simulink model "Rus_ver_model"  (R2021b)
settings: Solver=ode15s  StartTime=0.0  StopTime=10  FixedStep=1e-2  MaxStep=tsTraj  RelTol=1e-3  EnableMultiTasking=on
values from neighbouring files (symbols this model uses):
  bd_spine_damping = 0    [CostFcnPDcontroll.m]    (also in CostFuncOptimizeSpine.m = spine_param(3); last_scores.mat = 10)
  bd_spine_eq_pos = 0    [CostFcnPDcontroll.m]    (also in CostFuncOptimizeSpine.m = deg2rad(spine_param(1)); last_scores.mat)
  bd_spine_stiffness = 0    [CostFcnPDcontroll.m]    (also in CostFuncOptimizeSpine.m = spine_param(2); last_scores.mat = 300)
  body_dim = [0.267 0.194 0.114]    [last_scores.mat]    (also in robotParameters.m)
  body_mass = 6.0    (= 6)    [CostOfTransport.m]    (also in last_scores.mat; robotParameters.m)
  delta_gait_front = delays(1)    [CostFuncOptimizeSpine.m]    (also in PD_optimizedData_16Mar22_1632.mat = 48; PD_optimizedData_16Mar22_2228_good.mat = 58; PD_optimizedData_17Mar22_1432_vel_walk_03735.mat = 56; PD_optimizedData_18Mar22_1518_right_direction.mat = 46)
  delta_gait_rear = delays(2)    [CostFuncOptimizeSpine.m]    (also in PD_optimizedData_16Mar22_1632.mat = 56; PD_optimizedData_16Mar22_2228_good.mat = 40; PD_optimizedData_17Mar22_1432_vel_walk_03735.mat = 6; PD_optimizedData_18Mar22_1518_right_direction.mat = 76)
  fem_der_front = [0 1.0471975512 -3.66519142919 -6.45771823238 -0.523598775598 5.41052068118 0]    [last_scores.mat]
  fem_der_rear = [0 -2.61799387799 -0.872664625997 1.2217304764 4.88692190558 1.3962634016 0]    [last_scores.mat]
  fem_motionFront = femur_motionFront    [CostFcnPDcontroll.m]    (also in CostFuncOptimizeSpine.m = deg2rad([params(1:N), params(1)]); getFiguresAngOmTau.m; last_scores.mat = [-2.12930168743 -2.33874119767 -2.26892802759 -2.12930168743; nonlinearContraints.m = deg2rad([x(1:N), x(1)]))
  fem_motionRear = femur_motionRear    [CostFcnPDcontroll.m]    (also in CostFuncOptimizeSpine.m = deg2rad([params(2*N+1:3*N), params(2*N+1)]); getFiguresAngOmTau.m; last_scores.mat = [-2.09439510239 -2.12930168743 -2.16420827247 -2.19911485751; nonlinearContraints.m = deg2rad([x(2*N+1:3*N), x(2*N+1)]))
  gait_period = 1.2    [PD_optimizedData_16Mar22_1632.mat]    (also in PD_optimizedData_16Mar22_2228_good.mat; PD_optimizedData_17Mar22_1432_vel_walk_03735.mat; PD_optimizedData_18Mar22_1518_right_direction.mat; PD_optimizedData_18Mar22_1539.mat)
  ground = [20 2 0.1]    [last_scores.mat]    (also in robotParameters.m = [20 1.5 0.05])
  hip_mass = 0.595    [CostOfTransport.m]    (also in last_scores.mat; robotParameters.m)
  hip_radius = 0.046    [last_scores.mat]    (also in robotParameters.m)
  max_torque = 33.5    [last_scores.mat]    (also in robotParameters.m)
  N = (numel(params)-5)/4    [CostFuncOptimizeSpine.m]    (also in nonlinearContraints.m = (numel(x)-2)/4; nonlinearContraintsSpine.m = (numel(x)-5)/4; pampam.m = numel(params)/2)
  tib_der_front = [0 -1.74532925199 0.349065850399 0 1.57079632679 1.74532925199 0]    [last_scores.mat]
  tib_der_rear = [0 0.698131700798 -1.3962634016 3.31612557879 2.44346095279 -4.01425727959 0]    [last_scores.mat]
  tib_motionFront = tibia_motionFront    [CostFcnPDcontroll.m]    (also in CostFuncOptimizeSpine.m = deg2rad([params(N+1:2*N), params(N+1)]); getFiguresAngOmTau.m; last_scores.mat = [1.0471975512 0.977384381117 0.872664625997 0.977384381117 1; nonlinearContraints.m = deg2rad([x(N+1:2*N), x(N+1)]))
  tib_motionRear = tibia_motionRear    [CostFcnPDcontroll.m]    (also in CostFuncOptimizeSpine.m = deg2rad([params(3*N+1:4*N), params(3*N+1)]); getFiguresAngOmTau.m; last_scores.mat = [0.942477796077 1.08210413624 0.733038285838 1.18682389136 1; nonlinearContraints.m = deg2rad([x(3*N+1:4*N), x(3*N+1)]))
  traj_times = linspace(0,gait_period,N+1)    [CostFuncOptimizeSpine.m]    (also in PD_optimizedData_16Mar22_1632.mat = [0 0.2 0.4 0.6 0.8 1 1.2]; PD_optimizedData_16Mar22_2228_good.mat = [0 0.2 0.4 0.6 0.8 1 1.2]; PD_optimizedData_17Mar22_1432_vel_walk_03735.mat = [0 0.2 0.4 0.6 0.8 1 1.2]; PD_optimizedData_18Mar22_1518_right_direction.mat = [0 0.2 0.4 0.6 0.8 1 1.2])
  tsTraj = 0.01    [last_scores.mat]    (also in pampam.m; robotParameters.m)
undefined symbols (not defined in the file or in its folder): X, Y, Z
libraries: sm_lib x72, simulink x12, nesl_utility x10, robotcorelib x4, QR_leg_rus_ver x4
(part 1 of 3)
settings Model: SimulationMode=accelerator  Creator=boris_1863  LastModifiedBy=YEfim
settings SolverCC: AlgebraicLoopSolver=TrustRegion  SolverResetMethod=Robust
settings DataIOCC: LimitDataPoints=on  MaxDataPoints=10000
settings OptimizationCC: LifeSpan=inf
settings DebuggingCC: IgnoredZcDiagnostic=none  AllowSymbolicDim=off  SFUnexpectedBacktrackingDiag=warning  SFNoUnconditionalDefaultTransitionDiag=warning  SFExecutionAtInitializationDiag=none  SFMachineParentedDataDiag=warning  ArithmeticOperatorsInVariantConditions=warning
settings HardwareCC: ProdBitPerLong=64  ProdHWDeviceType=Intel->x86-64 (Linux 64)
settings SFSimCC: SimUseLocalCustomCode=off  CustomCodeUndefinedFunction=UseInterfaceOnly
settings RTWCC: RTWUseLocalCustomCode=off
settings CodeAppCC: StateflowObjectComments=on
settings GRTTargetCC: TargetLangStandard=C89/C90 (ANSI)
settings ConfigComp: CovMetricSettings=dw  CovSaveCumulativeToWorkspaceVar=on  CovSaveSingleToWorkspaceVar=on  CovExternalEMLEnable=off  CovSFcnEnable=off
settings SimscapeCC: SimscapeNormalizeSystem=off  SimscapeLogDataHistory=10000
settings DiagnosticsConfigSet: SimMechanicsInvalidVisualProperty=none  SimMechanicsCrossSectionNullEdge=none  SimMechanicsUnconnectedFramePorts=none  SimMechanicsUnconnectedGeometryPorts=none  SimMechanicsRedundantBlock=none  SimMechanicsConflictingReferenceFrames=none  SimMechanicsRigidlyBoundBlock=none  SimMechanicsUnsatisfiedHighPriorityTargets=none  SimMechanicsJointTargetOverSpecification=none
settings ExplorerConfigSet: InternalSimMechanicsExplorerSettings="<ExplorerConfiguration><canonicalview>default</canonicalview><AnimationSetting><BasePlaybackSpeed>1.0</BasePlaybackSpeed><PlaybackSpeedFactor>0.5</PlaybackSpeedFactor></AnimationSetting><TilePanel><TileInfo><Tiles Columns=\"1\" Count=\"1\" Rows=\"1\"><Column Weight=\"1\"/><Row Weight=\"1\"/><Tile Height=\"1\" Width=\"1\" X=\"0\" Y=\"0\"/></Tiles></TileInfo><SceneInfo><SceneViewer><BGColor><R>1</R><G>1</G><B>1</B></BGColor><Camera><DoPerspective>off</DoPerspective><Position><X>2.30591075274786395</X><Y>-10.1183993179019129</Y><Z>0.217589827418119802</Z></Position><Center><X>2.30591075274786395</X><Y>3.02154239351093423e-07</Y><Z>0.217589827418119802</Z></Center><Up><X>0</X><Y>-0</Y><Z>1</Z></Up><ViewLimDist>1</ViewLimDist><YLim>0.757338786635555206</YLim><XLim>2.71140067704754673</XLim></Camera></SceneViewer></SceneInfo></TilePanel><MechEditorPanel><Cameras/><GfxPanelCameraMap/><VideoCreator><PlaybackSpeedRatio>1.0</PlaybackSpeedRatio><FrameRate>60</FrameRate><VideoFormat>Motion JPEG AVI</VideoFormat><FrameSize>auto</FrameSize></VideoCreator></MechEditorPanel></ExplorerConfiguration>"

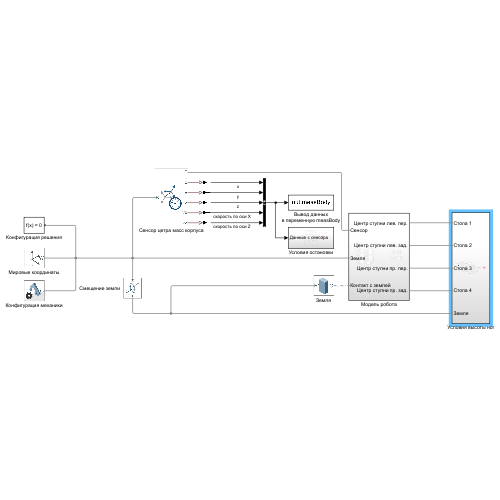
[thumbnail: Simulink's stored preview of the top-level diagram]
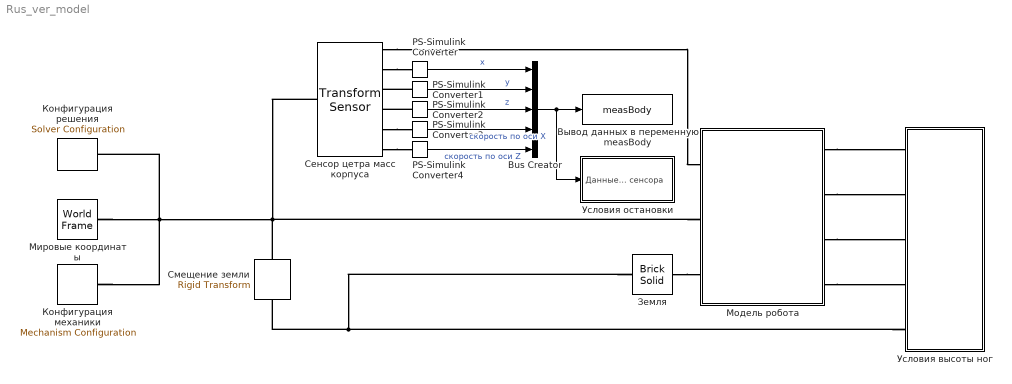
== system Rus_ver_model ==
  Bus Creator : BusCreator  Inputs=5
  PS-Simulink Converter : nesl_utility/PS-Simulink Converter  PhysicalDomain=network_engine_domain  SubClassName=ps_output  LeftPortType=input  RightPortType=output  PseudoPeriodic=off  Frequencies=[]  Unit=m  AffineConversion=off
      settings: SourceProductBaseCode=PW,SS
  PS-Simulink Converter1 : nesl_utility/PS-Simulink Converter  PhysicalDomain=network_engine_domain  SubClassName=ps_output  LeftPortType=input  RightPortType=output  PseudoPeriodic=off  Frequencies=[]  Unit=m  AffineConversion=off
      settings: SourceProductBaseCode=PW,SS
  PS-Simulink Converter2 : nesl_utility/PS-Simulink Converter  PhysicalDomain=network_engine_domain  SubClassName=ps_output  LeftPortType=input  RightPortType=output  PseudoPeriodic=off  Frequencies=[]  Unit=m  AffineConversion=off
      settings: SourceProductBaseCode=PW,SS
  PS-Simulink Converter3 : nesl_utility/PS-Simulink Converter  PhysicalDomain=network_engine_domain  SubClassName=ps_output  LeftPortType=input  RightPortType=output  PseudoPeriodic=off  Frequencies=[]  Unit=m/s  AffineConversion=off
      settings: SourceProductBaseCode=PW,SS
  PS-Simulink Converter4 : nesl_utility/PS-Simulink Converter  PhysicalDomain=network_engine_domain  SubClassName=ps_output  LeftPortType=input  RightPortType=output  PseudoPeriodic=off  Frequencies=[]  Unit=m/s  AffineConversion=off
      settings: SourceProductBaseCode=PW,SS
  Вывод данных в переменную measBody : ToWorkspace  VariableName=measBody  SaveFormat=Timeseries  SampleTime=-1
  Земля : sm_lib/Body Elements/Brick Solid  GraphicAmbientColor=[0.15 0.15 0.15 1.0]  BasedOnType=Density  BrickDimensions=ground  BrickDimensionUnits=m  CenterOfMass=[0 0 0]  CenterOfMassUnits=m  GraphicDiffuseColor=[0.5 0.5 0.5]  Density=1000  DensityUnits=kg/m^3  DoExposeReferenceFrame=off  GraphicEmissiveColor=[0.0 0.0 0.0 1.0]  ExportEntireGeometry=on  SerializedFrames=<Frames><Frame><Id>Frame1</Id><Value><Name>F1</Name><Origin><Source>GeometricFeature</Source><FeatureName>+z surface</FeatureName></Origin><PrimaryAxis><DefinedDirection>+Z</DefinedDirection><Source>ReferenceFrame</Source><SourceDirection>+Z</SourceDirection><FeatureName></FeatureName></PrimaryAxis><SecondaryAxis><DefinedDirection>+X</DefinedDirection><Source>ReferenceFrame</Source><SourceDirection>+X</SourceDirection><FeatureName></FeatureName></SecondaryAxis></Value></Frame></Frames>  MarkerShape=Sphere  MarkerSize=10  GraphicType=FromGeometry  InertiaType=CalculateFromGeometry  Mass=1  MassUnits=kg  MomentsOfInertia=[1 1 1]  MomentsOfInertiaUnits=kg*m^2  GraphicOpacity=1.0  ProductsOfInertia=[0 0 0]  ProductsOfInertiaUnits=kg*m^2  GraphicShininess=75  GraphicSpecularColor=[0.5 0.5 0.5 1.0]  GraphicVisPropType=SimpleVisualProperties
  Конфигурация механики : sm_lib/Utilities/Mechanism Configuration  UniformGravity=Constant  GravityVector=[0 0 -9.80665]  GravityUnits=m/s^2  LinearizationDelta=0.001  JointModeTransitionNonlinearIterations=2
  Конфигурация решения : nesl_utility/Solver Configuration  PhysicalDomain=network_engine_domain  SubClassName=solver  LeftPortType=input  RightPortType=generic  Tones=[]  Harmonics=[]  SimulateNoise=off  Profile=off  UseLocalSampling=off  EnableSwitchedLinearOptims=on  FrequencyDomain=off  UseCCode=off  RelTol=0.001  AbsTol=1e-06  MinStep=1e-09  ToWorkspace=off  RevertToSquareIcSolve=off  NumHomotopyIterations=100  PhasorMode=off  PhasorModeNumHarmonics=1  DoDC=off  ResidualTolerance=1e-09  UseLocalSolver=off  LocalSolverChoice=NE_BACKWARD_EULER_ADVANCER  LocalSolverSampleTime=0.001  DoFixedCost=off  MaxNonlinIter=3  MaxModeIter=2  ComputeImpulses=off  ImpulseIterations=2  LinearAlgebra=Sparse  EquationFormulation=NE_TIME_EF  DelaysMemoryBudget=1024  AutomaticFiltering=on  FilteringTimeConstant=0.001  PartitionStorageMethod=AS_NEEDED  PartitionMemoryBudget=1024  PartitionMethod=FAST
      settings: SourceProductBaseCode=PW,SS
  Мировые координаты : sm_lib/Frames and Transforms/World Frame
  Модель робота : Subsystem
  Сенсор цетра масс корпуса : sm_lib/Frames and Transforms/Transform Sensor  MeasurementFrame=World  SenseAngle=off  SenseAxis=off  SenseAngle1=off  SenseAngle2=off  SenseAngle3=off  SenseQ=off  SenseR=off  SenseOmegaX=off  SenseOmegaY=off  SenseOmegaZ=off  SenseOmega1=off  SenseOmega2=off  SenseOmega3=off  SenseQDot=off  SenseRDot=off  SenseAlphaX=off  SenseAlphaY=off  SenseAlphaZ=off  SenseAlpha1=off  SenseAlpha2=off  SenseAlpha3=off  SenseQDDot=off  SenseRDDot=off  SenseX=on  SenseY=on  SenseZ=on  SenseRad=off  SenseAzim=off  SenseDist=off  SenseInc=off  SenseXDot=on  SenseYDot=off  SenseZDot=on  SenseRadDot=off  SenseAzimDot=off  SenseDistDot=off  SenseIncDot=off  SenseXDDot=off  SenseYDDot=off  SenseZDDot=off  SenseRadDDot=off  SenseAzimDDot=off  SenseDistDDot=off  SenseIncDDot=off
  Смещение земли : sm_lib/Frames and Transforms/Rigid Transform  TranslationMethod=StandardAxis  TranslationStandardOffset=ground(1)/2-2  TranslationLengthUnit=m  TranslationStandardAxis=+X  TranslationCartesianOffset=[0 0 0]  TranslationROffset=0  TranslationROffsetUnits=m  TranslationZOffset=0  TranslationZOffsetUnits=m  TranslationThetaOffset=0  TranslationThetaOffsetUnits=deg  RotationMethod=None  RotationAngleUnits=deg  RotationStandardAxis=+Z  RotationAngle=0.0  RotationArbitraryAxis=[0 0 1]  FollAlignAxisA=+X  BaseAlignAxisA=+Y  FollAlignAxisB=+Y  BaseAlignAxisB=+Z  RotationSequenceAxes=FollowerAxes  RotationSequence=XYX  RotationSequenceAngles=[0 0 0]  RotationSequenceAnglesUnits=deg  RotationMatrix=[1 0 0; 0 1 0; 0 0 1]
  Условия высоты ног : Subsystem
  Условия остановки : Subsystem
  wires:
  PS-Simulink Converter/1 -> Bus Creator/1  "x"
  PS-Simulink Converter1/1 -> Bus Creator/2  "y"
  PS-Simulink Converter2/1 -> Bus Creator/3  "z"
  Bus Creator/1 -> Вывод данных в переменную measBody/1, Условия остановки/1(Данные с сенсора)
  PS-Simulink Converter3/1 -> Bus Creator/4  "скорость по оси X"
  PS-Simulink Converter4/1 -> Bus Creator/5  "скорость по оси Z"
  connections:
  Мировые координаты/RConn1 -- Конфигурация решения/RConn1 -- Сенсор цетра масс корпуса/LConn1 -- Смещение земли/LConn1 -- Модель робота/LConn2 -- Конфигурация механики/RConn1
  Земля/LConn1 -- Условия высоты ног/RConn5 -- Смещение земли/RConn1
  Сенсор цетра масс корпуса/RConn1 -- Модель робота/LConn1
  Земля/RConn1 -- Модель робота/LConn3
  Модель робота/RConn1 -- Условия высоты ног/RConn1
  Модель робота/RConn2 -- Условия высоты ног/RConn2
  Модель робота/RConn3 -- Условия высоты ног/RConn3
  Модель робота/RConn4 -- Условия высоты ног/RConn4
  Сенсор цетра масс корпуса/RConn2 -- PS-Simulink Converter/LConn1
  PS-Simulink Converter1/LConn1 -- Сенсор цетра масс корпуса/RConn3
  PS-Simulink Converter2/LConn1 -- Сенсор цетра масс корпуса/RConn4
  Сенсор цетра масс корпуса/RConn5 -- PS-Simulink Converter3/LConn1
  Сенсор цетра масс корпуса/RConn6 -- PS-Simulink Converter4/LConn1

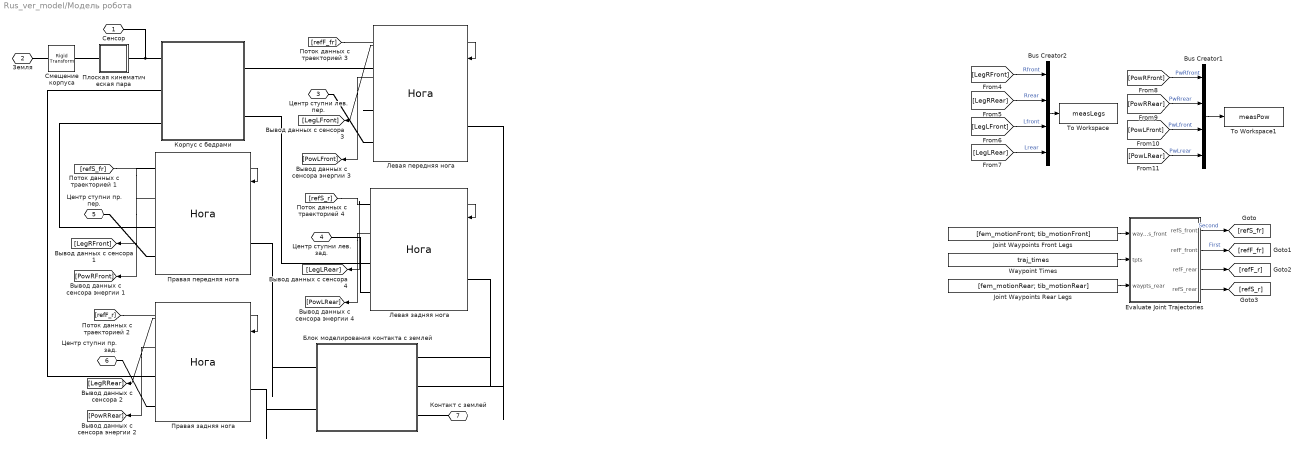
== system Rus_ver_model/Модель робота ==
  Bus Creator1 : BusCreator  Inputs=4
  Bus Creator2 : BusCreator  Inputs=4
  Evaluate Joint Trajectories : Subsystem
  Joint Waypoints Front Legs : Constant  Value=[fem_motionFront; tib_motionFront]
  Joint Waypoints Rear Legs : Constant  Value=[fem_motionRear; tib_motionRear]
  To Workspace : ToWorkspace  VariableName=measLegs  SaveFormat=Timeseries  SampleTime=-1
  To Workspace1 : ToWorkspace  VariableName=measPow  SaveFormat=Timeseries  SampleTime=-1
  Waypoint Times : Constant  Value=traj_times
  Блок моделирования контакта с землей : Subsystem
      settings: PortSchema="{\"entries\":[{\"content\":{\"sides\":[{\"content\":{\"connectorIds\":[]},\"type\":\"ConnectorPlacement.EquallySpacedRectSide\",\"uuid\":\"69850bd1-3a1b-4e19-820a-6c4fb91f3aa2\"},{\"content\":{\"connectorIds\":[],\"side\":\"RIGHT\"},\"type\":\"ConnectorPlacement.EquallySpacedRectSide\",\"uuid\":\"42ed8d47-3271-4e69-91e2-9f0454d59b48\"},{\"content\":{\"connectorIds\":[\"LConn1\",\"LConn2\"],\"side\":\"TOP\"},\"type\":\"ConnectorPlacement.EquallySpacedRectSide\",\"uuid\":\"114d7e17-c6c5-438c-9cb4-0dcf13920f6f\"},{\"content\":{\"connectorIds\":[\"RConn1\",\"RConn2\",\"RConn3\"],\"side\":\"BOTTOM\"},\"type\":\"ConnectorPlacement.EquallySpacedRectSide\",\"uuid\":\"caba5647-a516-4a04-8cbe-0248367597c4\"}]},\"type\":\"ConnectorPlacement.EquallySpacedConnector\",\"uuid\":\"24d64392-cc0c-4894-a6df-54d1d4435d86\"}],\"packageUris\":[\"http://schema.mathworks.com/mf0/Connector/R2020b\"],\"version\":\"1.0\"}"
  Корпус с бедрами : Subsystem  Variant=on  VariantControl=Choice  mask{spine_eq_pos=bd_spine_eq_pos, spine_stiffness=bd_spine_stiffness, spine_damping=bd_spine_damping}
      mask prompts: spine_eq_pos "Equilibrium Position"; spine_stiffness "Spring Stifness"; spine_damping "Damping Coefficient"
      mask DialogControl ParameterGroupVar Prompt: Spine's param
  Левая задняя нога : QR_leg_rus_ver/Нога  femur_l=0.13  tibia_l=0.18  leg_w=0.03  leg_w_t=0  qf_0=-135  qt_0=90  femur_cl=[0.2 0.2 1.0]  tibia_cl=[0.6 0.6 1.0]  kp_femur=k_p_fem  ki_femur=k_i_fem  kd_femur=k_d_fem  maxFemur=max_torque  minFemur=-max_torque  kp_tibia=k_p_tib  ki_tibia=k_i_tib  kd_tibia=k_d_tib  maxTibia=max_torque  minTibia=-max_torque  pwm_freq=PWM_freq  motor_voltage=m_voltage  motor_inductance=arm_inductance  motor_s_tau=stall_torque_motor  motor_nl_speed=no_load_speed_motor  motor_inertia=rotor_inertia  motor_damping=rotor_damping  gear_ratio=g_ratio
  Левая передняя нога : QR_leg_rus_ver/Нога  femur_l=0.13  tibia_l=0.18  leg_w=0.03  leg_w_t=0  qf_0=-135  qt_0=90  femur_cl=[0.2 0.2 1.0]  tibia_cl=[0.6 0.6 1.0]  kp_femur=k_p_fem  ki_femur=k_i_fem  kd_femur=k_d_fem  maxFemur=max_torque  minFemur=-max_torque  kp_tibia=k_p_tib  ki_tibia=k_i_tib  kd_tibia=k_d_tib  maxTibia=max_torque  minTibia=-max_torque  pwm_freq=PWM_freq  motor_voltage=m_voltage  motor_inductance=arm_inductance  motor_s_tau=stall_torque_motor  motor_nl_speed=no_load_speed_motor  motor_inertia=rotor_inertia  motor_damping=rotor_damping  gear_ratio=g_ratio
  Плоская кинематическая пара : Subsystem
  Правая задняя нога : QR_leg_rus_ver/Нога  femur_l=0.13  tibia_l=0.18  leg_w=0.03  leg_w_t=0  qf_0=-135  qt_0=90  femur_cl=[0.2 0.2 1.0]  tibia_cl=[0.6 0.6 1.0]  kp_femur=k_p_fem  ki_femur=k_i_fem  kd_femur=k_d_fem  maxFemur=max_torque  minFemur=-max_torque  kp_tibia=k_p_tib  ki_tibia=k_i_tib  kd_tibia=k_d_tib  maxTibia=max_torque  minTibia=-max_torque  pwm_freq=PWM_freq  motor_voltage=m_voltage  motor_inductance=arm_inductance  motor_s_tau=stall_torque_motor  motor_nl_speed=no_load_speed_motor  motor_inertia=rotor_inertia  motor_damping=rotor_damping  gear_ratio=g_ratio
  Правая передняя нога : QR_leg_rus_ver/Нога  femur_l=0.13  tibia_l=0.18  leg_w=0.03  leg_w_t=0  qf_0=-135  qt_0=90  femur_cl=[0.2 0.2 1.0]  tibia_cl=[0.6 0.6 1.0]  kp_femur=k_p_fem  ki_femur=k_i_fem  kd_femur=k_d_fem  maxFemur=max_torque  minFemur=-max_torque  kp_tibia=k_p_tib  ki_tibia=k_i_tib  kd_tibia=k_d_tib  maxTibia=max_torque  minTibia=-max_torque  pwm_freq=PWM_freq  motor_voltage=m_voltage  motor_inductance=arm_inductance  motor_s_tau=stall_torque_motor  motor_nl_speed=no_load_speed_motor  motor_inertia=rotor_inertia  motor_damping=rotor_damping  gear_ratio=g_ratio
  Смещение корпуса : sm_lib/Frames and Transforms/Rigid Transform  TranslationMethod=StandardAxis  TranslationStandardOffset=z_offset  TranslationLengthUnit=m  TranslationStandardAxis=+Z  TranslationCartesianOffset=[0 0 0]  TranslationROffset=0  TranslationROffsetUnits=m  TranslationZOffset=0  TranslationZOffsetUnits=m  TranslationThetaOffset=0  TranslationThetaOffsetUnits=deg  RotationMethod=None  RotationAngleUnits=deg  RotationStandardAxis=+Z  RotationAngle=0.0  RotationArbitraryAxis=[0 0 1]  FollAlignAxisA=+X  BaseAlignAxisA=+Y  FollAlignAxisB=+Y  BaseAlignAxisB=+Z  RotationSequenceAxes=FollowerAxes  RotationSequence=XYX  RotationSequenceAngles=[0 0 0]  RotationSequenceAnglesUnits=deg  RotationMatrix=[1 0 0; 0 1 0; 0 0 1]
  Сенсор : PMIOPort  Side=Left
  Земля : PMIOPort  Port=2  Side=Left
  Центр ступни лев. пер. : PMIOPort  Port=3  Side=Right
  Центр ступни лев. зад. : PMIOPort  Port=4  Side=Right
  Центр ступни пр. пер. : PMIOPort  Port=5  Side=Right
  Центр ступни пр. зад. : PMIOPort  Port=6  Side=Right
  Контакт с землей : PMIOPort  Port=7  Side=Left
  wires:
  [refF_r] -> Правая задняя нога/1
  Правая передняя нога/1 -> [LegRFront]
  Правая задняя нога/1 -> [LegRRear]
  Левая передняя нога/1 -> [LegLFront]
  Правая передняя нога/2 -> [PowRFront]
  Левая задняя нога/1 -> [LegLRear]
  [refS_fr] -> Правая передняя нога/1
  Правая задняя нога/2 -> [PowRRear]
  Левая задняя нога/2 -> [PowLRear]
  [refF_fr] -> Левая передняя нога/1
  Левая передняя нога/2 -> [PowLFront]
  [refS_r] -> Левая задняя нога/1
  Joint Waypoints Rear Legs/1 -> Evaluate Joint Trajectories/3(waypts_rear)
  Evaluate Joint Trajectories/1(refS_front) -> [refS_fr]  "Second"
  Evaluate Joint Trajectories/4(refS_rear) -> [refS_r]
  Evaluate Joint Trajectories/2(refF_front) -> [refF_fr]  "First"
  Joint Waypoints Front Legs/1 -> Evaluate Joint Trajectories/1(waypts_front)
  Waypoint Times/1 -> Evaluate Joint Trajectories/2(tpts)
  Evaluate Joint Trajectories/3(refF_rear) -> [refF_r]
  Bus Creator1/1 -> To Workspace1/1
  [PowLFront] -> Bus Creator1/3  "PwLfront"
  [PowRRear] -> Bus Creator1/2  "PwRrear"
  [PowRFront] -> Bus Creator1/1  "PwRfront"
  [LegLFront] -> Bus Creator2/3  "Lfront"
  [LegLRear] -> Bus Creator2/4  "Lrear"
  [LegRFront] -> Bus Creator2/1  "Rfront"
  [LegRRear] -> Bus Creator2/2  "Rrear"
  Bus Creator2/1 -> To Workspace/1
  [PowLRear] -> Bus Creator1/4  "PwLrear"
  connections:
  Левая задняя нога/RConn1 -- Корпус с бедрами/RConn2
  Правая задняя нога/RConn2 -- Центр ступни пр. зад./RConn1
  Левая передняя нога/RConn2 -- Центр ступни лев. пер./RConn1
  Правая задняя нога/RConn1 -- Корпус с бедрами/LConn2
  Левая передняя нога/RConn1 -- Корпус с бедрами/RConn1
  Корпус с бедрами/LConn1 -- Плоская кинематическая пара/RConn1 -- Сенсор/RConn1
  Правая передняя нога/RConn1 -- Корпус с бедрами/LConn3
  Плоская кинематическая пара/LConn1 -- Смещение корпуса/RConn1
  Левая задняя нога/RConn2 -- Центр ступни лев. зад./RConn1
  Правая передняя нога/RConn2 -- Центр ступни пр. пер./RConn1
  Смещение корпуса/LConn1 -- Земля/RConn1
  Правая задняя нога/LConn1 -- Блок моделирования контакта с землей/LConn1
  Блок моделирования контакта с землей/RConn1 -- Контакт с землей/RConn1
  Левая задняя нога/LConn1 -- Блок моделирования контакта с землей/RConn3
  Левая передняя нога/LConn1 -- Блок моделирования контакта с землей/RConn2
  Правая передняя нога/LConn1 -- Блок моделирования контакта с землей/LConn2

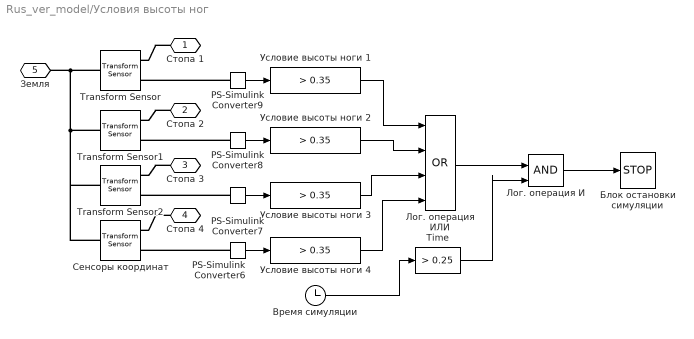
== system Rus_ver_model/Условия высоты ног ==
  PS-Simulink Converter{6..9} (4 alike) : nesl_utility/PS-Simulink Converter  PhysicalDomain=network_engine_domain  SubClassName=ps_output  LeftPortType=input  RightPortType=output  PseudoPeriodic=off  Frequencies=[]  Unit=inherit  AffineConversion=off
      settings: SourceProductBaseCode=PW,SS
  "Time " : simulink/Logic and Bit Operations/Compare To Constant  relop=>  const=0.25  OutDataTypeStr=boolean
  Transform Sensor : sm_lib/Frames and Transforms/Transform Sensor  MeasurementFrame=Base  SenseAngle=off  SenseAxis=off  SenseAngle1=off  SenseAngle2=off  SenseAngle3=off  SenseQ=off  SenseR=off  SenseOmegaX=off  SenseOmegaY=off  SenseOmegaZ=off  SenseOmega1=off  SenseOmega2=off  SenseOmega3=off  SenseQDot=off  SenseRDot=off  SenseAlphaX=off  SenseAlphaY=off  SenseAlphaZ=off  SenseAlpha1=off  SenseAlpha2=off  SenseAlpha3=off  SenseQDDot=off  SenseRDDot=off  SenseX=off  SenseY=off  SenseZ=on  SenseRad=off  SenseAzim=off  SenseDist=off  SenseInc=off  SenseXDot=off  SenseYDot=off  SenseZDot=off  SenseRadDot=off  SenseAzimDot=off  SenseDistDot=off  SenseIncDot=off  SenseXDDot=off  SenseYDDot=off  SenseZDDot=off  SenseRadDDot=off  SenseAzimDDot=off  SenseDistDDot=off  SenseIncDDot=off
  Transform Sensor1 : sm_lib/Frames and Transforms/Transform Sensor  MeasurementFrame=Base  SenseAngle=off  SenseAxis=off  SenseAngle1=off  SenseAngle2=off  SenseAngle3=off  SenseQ=off  SenseR=off  SenseOmegaX=off  SenseOmegaY=off  SenseOmegaZ=off  SenseOmega1=off  SenseOmega2=off  SenseOmega3=off  SenseQDot=off  SenseRDot=off  SenseAlphaX=off  SenseAlphaY=off  SenseAlphaZ=off  SenseAlpha1=off  SenseAlpha2=off  SenseAlpha3=off  SenseQDDot=off  SenseRDDot=off  SenseX=off  SenseY=off  SenseZ=on  SenseRad=off  SenseAzim=off  SenseDist=off  SenseInc=off  SenseXDot=off  SenseYDot=off  SenseZDot=off  SenseRadDot=off  SenseAzimDot=off  SenseDistDot=off  SenseIncDot=off  SenseXDDot=off  SenseYDDot=off  SenseZDDot=off  SenseRadDDot=off  SenseAzimDDot=off  SenseDistDDot=off  SenseIncDDot=off
  Transform Sensor2 : sm_lib/Frames and Transforms/Transform Sensor  MeasurementFrame=Base  SenseAngle=off  SenseAxis=off  SenseAngle1=off  SenseAngle2=off  SenseAngle3=off  SenseQ=off  SenseR=off  SenseOmegaX=off  SenseOmegaY=off  SenseOmegaZ=off  SenseOmega1=off  SenseOmega2=off  SenseOmega3=off  SenseQDot=off  SenseRDot=off  SenseAlphaX=off  SenseAlphaY=off  SenseAlphaZ=off  SenseAlpha1=off  SenseAlpha2=off  SenseAlpha3=off  SenseQDDot=off  SenseRDDot=off  SenseX=off  SenseY=off  SenseZ=on  SenseRad=off  SenseAzim=off  SenseDist=off  SenseInc=off  SenseXDot=off  SenseYDot=off  SenseZDot=off  SenseRadDot=off  SenseAzimDot=off  SenseDistDot=off  SenseIncDot=off  SenseXDDot=off  SenseYDDot=off  SenseZDDot=off  SenseRadDDot=off  SenseAzimDDot=off  SenseDistDDot=off  SenseIncDDot=off
  Блок остановки симуляции : Stop
  Время симуляции : Clock
  Лог. операция И : Logic  IconShape=distinctive  AllPortsSameDT=off  OutDataTypeStr=boolean
  Лог. операция ИЛИ : Logic  Operator=OR  Inputs=4  AllPortsSameDT=off  OutDataTypeStr=boolean
  Сенсоры координат : sm_lib/Frames and Transforms/Transform Sensor  MeasurementFrame=Base  SenseAngle=off  SenseAxis=off  SenseAngle1=off  SenseAngle2=off  SenseAngle3=off  SenseQ=off  SenseR=off  SenseOmegaX=off  SenseOmegaY=off  SenseOmegaZ=off  SenseOmega1=off  SenseOmega2=off  SenseOmega3=off  SenseQDot=off  SenseRDot=off  SenseAlphaX=off  SenseAlphaY=off  SenseAlphaZ=off  SenseAlpha1=off  SenseAlpha2=off  SenseAlpha3=off  SenseQDDot=off  SenseRDDot=off  SenseX=off  SenseY=off  SenseZ=on  SenseRad=off  SenseAzim=off  SenseDist=off  SenseInc=off  SenseXDot=off  SenseYDot=off  SenseZDot=off  SenseRadDot=off  SenseAzimDot=off  SenseDistDot=off  SenseIncDot=off  SenseXDDot=off  SenseYDDot=off  SenseZDDot=off  SenseRadDDot=off  SenseAzimDDot=off  SenseDistDDot=off  SenseIncDDot=off
  Условие высоты ноги {1..4} (4 alike) : simulink/Logic and Bit Operations/Compare To Constant  relop=>  const=0.35  OutDataTypeStr=boolean
  Стопа 1 : PMIOPort  Side=Right
  Стопа 2 : PMIOPort  Port=2  Side=Right
  Стопа 3 : PMIOPort  Port=3  Side=Right
  Стопа 4 : PMIOPort  Port=4  Side=Right
  Земля : PMIOPort  Port=5  Side=Right
  wires:
  PS-Simulink Converter6/1 -> Условие высоты ноги 4/1
  Лог. операция ИЛИ/1 -> Лог. операция И/1
  PS-Simulink Converter7/1 -> Условие высоты ноги 3/1
  Время симуляции/1 -> "Time "/1
  PS-Simulink Converter9/1 -> Условие высоты ноги 1/1
  PS-Simulink Converter8/1 -> Условие высоты ноги 2/1
  Условие высоты ноги 2/1 -> Лог. операция ИЛИ/2
  Условие высоты ноги 4/1 -> Лог. операция ИЛИ/4
  "Time "/1 -> Лог. операция И/2
  Условие высоты ноги 3/1 -> Лог. операция ИЛИ/3
  Лог. операция И/1 -> Блок остановки симуляции/1
  Условие высоты ноги 1/1 -> Лог. операция ИЛИ/1
  connections:
  PS-Simulink Converter9/LConn1 -- Transform Sensor/RConn2
  PS-Simulink Converter8/LConn1 -- Transform Sensor1/RConn2
  Сенсоры координат/LConn1 -- Transform Sensor2/LConn1 -- Transform Sensor1/LConn1 -- Transform Sensor/LConn1 -- Земля/RConn1
  PS-Simulink Converter6/LConn1 -- Сенсоры координат/RConn2
  PS-Simulink Converter7/LConn1 -- Transform Sensor2/RConn2
  Стопа 3/RConn1 -- Transform Sensor2/RConn1
  Стопа 4/RConn1 -- Сенсоры координат/RConn1
  Стопа 2/RConn1 -- Transform Sensor1/RConn1
  Стопа 1/RConn1 -- Transform Sensor/RConn1

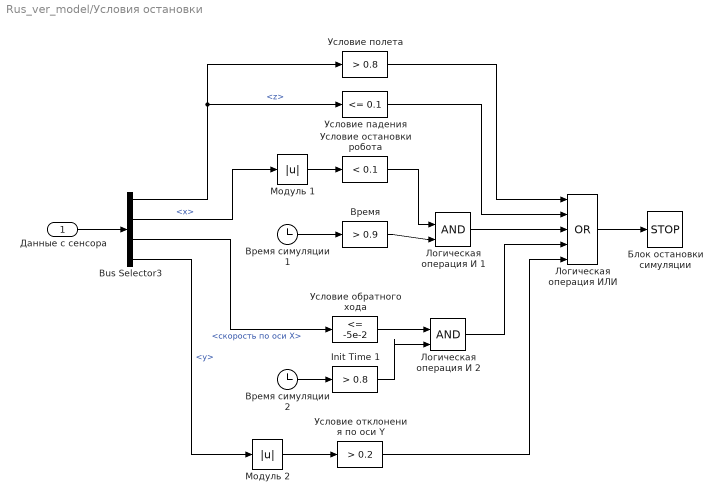
== system Rus_ver_model/Условия остановки ==
  Данные с сенсора : Inport
  Bus Selector3 : BusSelector  OutputSignals=z,x,скорость по оси X,y
  Init Time 1 : simulink/Logic and Bit Operations/Compare To Constant  relop=>  const=0.8  OutDataTypeStr=boolean
  Блок остановки симуляции : Stop
  Время симуляции 1 : Clock
  Время симуляции 2 : Clock
  "Время " : simulink/Logic and Bit Operations/Compare To Constant  relop=>  const=0.9  OutDataTypeStr=boolean
  Логическая операция И 1 : Logic  IconShape=distinctive  AllPortsSameDT=off  OutDataTypeStr=boolean
  Логическая операция ИЛИ : Logic  Operator=OR  Inputs=5  AllPortsSameDT=off  OutDataTypeStr=boolean
  Логическая операция И 2 : Logic  IconShape=distinctive  AllPortsSameDT=off  OutDataTypeStr=boolean
  Модуль 1 : Abs
  Модуль 2 : Abs
  Условие обратного хода : simulink/Logic and Bit Operations/Compare To Constant  relop=<=  const=-5e-2  OutDataTypeStr=boolean
  Условие остановки робота : simulink/Logic and Bit Operations/Compare To Constant  relop=<  const=0.1  OutDataTypeStr=boolean
  Условие отклонения по оси Y : simulink/Logic and Bit Operations/Compare To Constant  relop=>  const=0.2  OutDataTypeStr=boolean
  Условие падения : simulink/Logic and Bit Operations/Compare To Constant  relop=<=  const=0.1  OutDataTypeStr=boolean
  Условие полета : simulink/Logic and Bit Operations/Compare To Constant  relop=>  const=0.8  OutDataTypeStr=boolean
  wires:
  Условие падения/1 -> Логическая операция ИЛИ/2
  Данные с сенсора/1 -> Bus Selector3/1
  Bus Selector3/1 -> Условие полета/1, Условие падения/1  "<z>"
  Логическая операция ИЛИ/1 -> Блок остановки симуляции/1
  Условие полета/1 -> Логическая операция ИЛИ/1
  Bus Selector3/2 -> Модуль 1/1  "<x>"
  Условие остановки робота/1 -> Логическая операция И 1/1
  Модуль 1/1 -> Условие остановки робота/1
  Время симуляции 1/1 -> "Время "/1
  "Время "/1 -> Логическая операция И 1/2
  Логическая операция И 1/1 -> Логическая операция ИЛИ/3
  Bus Selector3/3 -> Условие обратного хода/1  "<скорость по оси X>"
  Время симуляции 2/1 -> Init Time 1/1
  Init Time 1/1 -> Логическая операция И 2/2
  Условие обратного хода/1 -> Логическая операция И 2/1
  Логическая операция И 2/1 -> Логическая операция ИЛИ/4
  Bus Selector3/4 -> Модуль 2/1  "<y>"
  Модуль 2/1 -> Условие отклонения по оси Y/1
  Условие отклонения по оси Y/1 -> Логическая операция ИЛИ/5

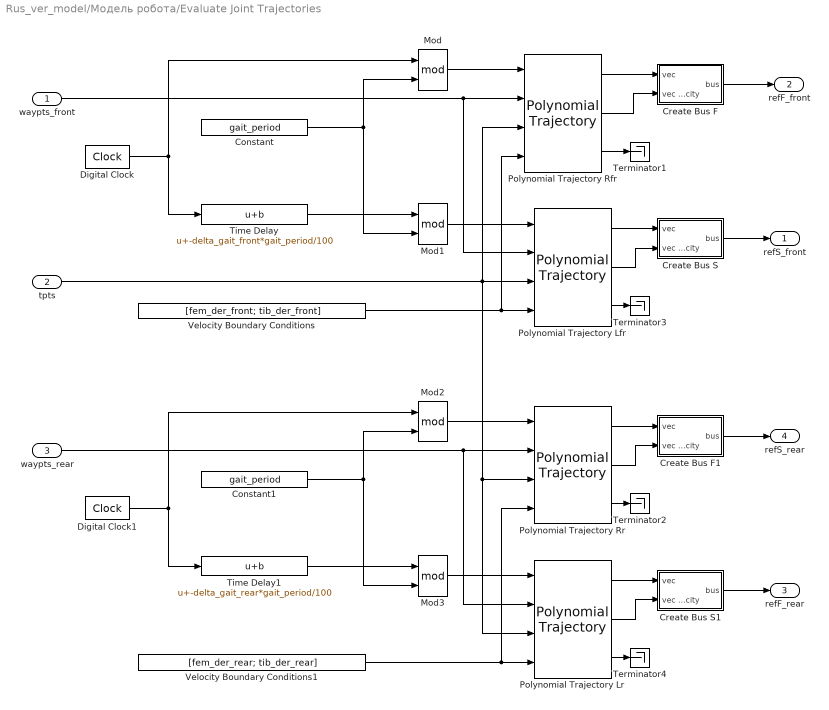
== system Rus_ver_model/Модель робота/Evaluate Joint Trajectories ==
  waypts_front : Inport
  tpts : Inport  Port=2
  waypts_rear : Inport  Port=3
  Constant : Constant  Value=gait_period
  Constant1 : Constant  Value=gait_period
  Create Bus F : Subsystem
  Create Bus F1 : Subsystem
  Create Bus S : Subsystem
  Create Bus S1 : Subsystem
  Digital Clock : DigitalClock  SampleTime=tsTraj
  Digital Clock1 : DigitalClock  SampleTime=tsTraj
  Mod{,1..3} (4 alike) : Math  Operator=mod  SaturateOnIntegerOverflow=on
  Polynomial Trajectory Lfr : robotcorelib/Polynomial Trajectory  WaypointSource=External  Waypoints=[ 0, 2, 1, 5, 0; -1, 3, 1, 4, 4 ]  TimePoints=[ 0, 1, 2, 3, 4 ]  TimeInterval=[ 1, 4 ]  Method=Cubic Polynomial  ParameterSource=External  VelocityBoundaryCondition=zeros( 2, 5 )  AccelerationBoundaryCondition=zeros( 2, 5 )  SimulateUsing=Interpreted execution
  Polynomial Trajectory Lr : robotcorelib/Polynomial Trajectory  WaypointSource=External  Waypoints=[ 0, 2, 1, 5, 0; -1, 3, 1, 4, 4 ]  TimePoints=[ 0, 1, 2, 3, 4 ]  TimeInterval=[ 1, 4 ]  Method=Cubic Polynomial  ParameterSource=External  VelocityBoundaryCondition=zeros( 2, 5 )  AccelerationBoundaryCondition=zeros( 2, 5 )  SimulateUsing=Interpreted execution
  Polynomial Trajectory Rfr : robotcorelib/Polynomial Trajectory  WaypointSource=External  Waypoints=[ 0, 2, 1, 5, 0; -1, 3, 1, 4, 4 ]  TimePoints=[ 0, 1, 2, 3, 4 ]  TimeInterval=[ 1, 4 ]  Method=Cubic Polynomial  ParameterSource=External  VelocityBoundaryCondition=zeros( 2, 5 )  AccelerationBoundaryCondition=zeros( 2, 5 )  SimulateUsing=Interpreted execution
  Polynomial Trajectory Rr : robotcorelib/Polynomial Trajectory  WaypointSource=External  Waypoints=[ 0, 2, 1, 5, 0; -1, 3, 1, 4, 4 ]  TimePoints=[ 0, 1, 2, 3, 4 ]  TimeInterval=[ 1, 4 ]  Method=Cubic Polynomial  ParameterSource=External  VelocityBoundaryCondition=zeros( 2, 5 )  AccelerationBoundaryCondition=zeros( 2, 5 )  SimulateUsing=Interpreted execution
  Terminator{1..4} (4 alike) : Terminator
  Time Delay : Bias  Bias=-delta_gait_front*gait_period/100
  Time Delay1 : Bias  Bias=-delta_gait_rear*gait_period/100
  Velocity Boundary Conditions : Constant  Value=[fem_der_front; tib_der_front]
  Velocity Boundary Conditions1 : Constant  Value=[fem_der_rear; tib_der_rear]
  refS_front : Outport
  refF_front : Outport  Port=2
  refF_rear : Outport  Port=3
  refS_rear : Outport  Port=4
  wires:
  Polynomial Trajectory Rfr/1 -> Create Bus F/1(vec)
  Create Bus S/1(bus) -> refS_front/1
  Create Bus F/1(bus) -> refF_front/1
  Polynomial Trajectory Lfr/1 -> Create Bus S/1(vec)
  Polynomial Trajectory Lfr/3 -> Terminator3/1
  Polynomial Trajectory Rfr/2 -> Create Bus F/2(vec velocity)
  Polynomial Trajectory Rfr/3 -> Terminator1/1
  Polynomial Trajectory Lfr/2 -> Create Bus S/2(vec velocity)
  Digital Clock/1 -> Mod/1, Time Delay/1
  waypts_front/1 -> Polynomial Trajectory Rfr/2, Polynomial Trajectory Lfr/2
  Velocity Boundary Conditions/1 -> Polynomial Trajectory Rfr/4, Polynomial Trajectory Lfr/4
  Mod/1 -> Polynomial Trajectory Rfr/1
  Mod1/1 -> Polynomial Trajectory Lfr/1
  Constant/1 -> Mod1/2, Mod/2
  Time Delay/1 -> Mod1/1
  Time Delay1/1 -> Mod3/1
  Constant1/1 -> Mod2/2, Mod3/2
  Mod3/1 -> Polynomial Trajectory Lr/1
  Mod2/1 -> Polynomial Trajectory Rr/1
  Velocity Boundary Conditions1/1 -> Polynomial Trajectory Rr/4, Polynomial Trajectory Lr/4
  tpts/1 -> Polynomial Trajectory Rfr/3, Polynomial Trajectory Lfr/3, Polynomial Trajectory Rr/3, Polynomial Trajectory Lr/3
  waypts_rear/1 -> Polynomial Trajectory Rr/2, Polynomial Trajectory Lr/2
  Digital Clock1/1 -> Time Delay1/1, Mod2/1
  Polynomial Trajectory Lr/2 -> Create Bus S1/2(vec velocity)
  Polynomial Trajectory Rr/3 -> Terminator2/1
  Polynomial Trajectory Rr/2 -> Create Bus F1/2(vec velocity)
  Polynomial Trajectory Lr/3 -> Terminator4/1
  Polynomial Trajectory Lr/1 -> Create Bus S1/1(vec)
  Create Bus F1/1(bus) -> refS_rear/1
  Create Bus S1/1(bus) -> refF_rear/1
  Polynomial Trajectory Rr/1 -> Create Bus F1/1(vec)

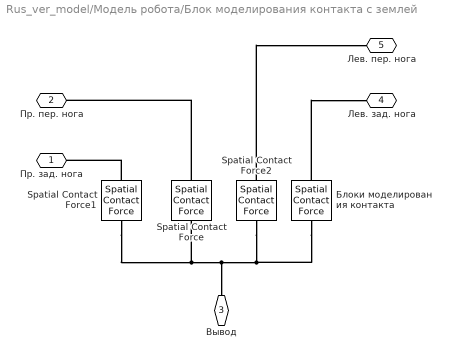
== system Rus_ver_model/Модель робота/Блок моделирования контакта с землей ==
  Spatial Contact Force : sm_lib/Forces and Torques/Spatial Contact Force  CoefficientOfDynamicFriction=dynamicFriction  CoefficientOfStaticFriction=staticFriction  SenseContactBaseRotation=off  SenseContactBaseTranslation=off  NormalDamping=cntdmp  NormalDampingUnits=N/(m/s)  SenseContactFollowerRotation=off  SenseContactFollowerTranslation=off  SenseContactSignal=off  NormalStiffness=cntstiff  NormalStiffnessUnits=N/m  FrictionalCriticalVelocity=mu_vth  FrictionalCriticalVelocityUnits=m/s  ZeroCrossDetectContactStartAndEnd=off  FrictionType=SmoothStickSlip  SenseFrictionalForceMagnitude=off  SenseNormalForceMagnitude=off  NormalForceType=SmoothSpringDamper  SenseNormalVelocity=off  SenseSeparationDistance=off  SenseTangentialVelocity=off  SenseTangentialVelocityMagnitude=off  NormalTransitionRegionWidth=1e-3  NormalTransitionRegionWidthUnits=m
  Spatial Contact Force1 : sm_lib/Forces and Torques/Spatial Contact Force  CoefficientOfDynamicFriction=dynamicFriction  CoefficientOfStaticFriction=staticFriction  SenseContactBaseRotation=off  SenseContactBaseTranslation=off  NormalDamping=cntdmp  NormalDampingUnits=N/(m/s)  SenseContactFollowerRotation=off  SenseContactFollowerTranslation=off  SenseContactSignal=off  NormalStiffness=cntstiff  NormalStiffnessUnits=N/m  FrictionalCriticalVelocity=mu_vth  FrictionalCriticalVelocityUnits=m/s  ZeroCrossDetectContactStartAndEnd=off  FrictionType=SmoothStickSlip  SenseFrictionalForceMagnitude=off  SenseNormalForceMagnitude=off  NormalForceType=SmoothSpringDamper  SenseNormalVelocity=off  SenseSeparationDistance=off  SenseTangentialVelocity=off  SenseTangentialVelocityMagnitude=off  NormalTransitionRegionWidth=1e-3  NormalTransitionRegionWidthUnits=m
  Spatial Contact Force2 : sm_lib/Forces and Torques/Spatial Contact Force  CoefficientOfDynamicFriction=dynamicFriction  CoefficientOfStaticFriction=staticFriction  SenseContactBaseRotation=off  SenseContactBaseTranslation=off  NormalDamping=cntdmp  NormalDampingUnits=N/(m/s)  SenseContactFollowerRotation=off  SenseContactFollowerTranslation=off  SenseContactSignal=off  NormalStiffness=cntstiff  NormalStiffnessUnits=N/m  FrictionalCriticalVelocity=mu_vth  FrictionalCriticalVelocityUnits=m/s  ZeroCrossDetectContactStartAndEnd=off  FrictionType=SmoothStickSlip  SenseFrictionalForceMagnitude=off  SenseNormalForceMagnitude=off  NormalForceType=SmoothSpringDamper  SenseNormalVelocity=off  SenseSeparationDistance=off  SenseTangentialVelocity=off  SenseTangentialVelocityMagnitude=off  NormalTransitionRegionWidth=1e-3  NormalTransitionRegionWidthUnits=m
  Блоки моделирования контакта : sm_lib/Forces and Torques/Spatial Contact Force  CoefficientOfDynamicFriction=dynamicFriction  CoefficientOfStaticFriction=staticFriction  SenseContactBaseRotation=off  SenseContactBaseTranslation=off  NormalDamping=cntdmp  NormalDampingUnits=N/(m/s)  SenseContactFollowerRotation=off  SenseContactFollowerTranslation=off  SenseContactSignal=off  NormalStiffness=cntstiff  NormalStiffnessUnits=N/m  FrictionalCriticalVelocity=mu_vth  FrictionalCriticalVelocityUnits=m/s  ZeroCrossDetectContactStartAndEnd=off  FrictionType=SmoothStickSlip  SenseFrictionalForceMagnitude=off  SenseNormalForceMagnitude=off  NormalForceType=SmoothSpringDamper  SenseNormalVelocity=off  SenseSeparationDistance=off  SenseTangentialVelocity=off  SenseTangentialVelocityMagnitude=off  NormalTransitionRegionWidth=1e-3  NormalTransitionRegionWidthUnits=m
  Пр. зад. нога : PMIOPort  Side=Left
  Пр. пер. нога : PMIOPort  Port=2  Side=Left
  Вывод : PMIOPort  Port=3  Side=Right
  Лев. зад. нога : PMIOPort  Port=4  Side=Right
  Лев. пер. нога : PMIOPort  Port=5  Side=Right
  connections:
  Spatial Contact Force/LConn1 -- Пр. пер. нога/RConn1
  Spatial Contact Force1/RConn1 -- Вывод/RConn1 -- Блоки моделирования контакта/RConn1 -- Spatial Contact Force2/RConn1 -- Spatial Contact Force/RConn1
  Блоки моделирования контакта/LConn1 -- Лев. зад. нога/RConn1
  Spatial Contact Force2/LConn1 -- Лев. пер. нога/RConn1
  Spatial Contact Force1/LConn1 -- Пр. зад. нога/RConn1

== system Rus_ver_model/Модель робота/Корпус с бедрами ==
  Жесткий корпус : Subsystem  VariantControl=(typeBody == 1)
  Податливый корпус : Subsystem  VariantControl=(typeBody == 2)
  Земля : PMIOPort  Side=Left
  Пр. зад. нога : PMIOPort  Port=2  Side=Left
  Лев. пер. нога : PMIOPort  Port=3  Side=Right
  Пр. пер. нога : PMIOPort  Port=4  Side=Left
  Лев. зад. нога : PMIOPort  Port=5  Side=Right
